simulink model "B737_PLANT"  (R2018a)
settings: Solver=VariableStepAuto  StartTime=0.0  StopTime=10.0  RelTol=1e-3
undefined symbols (not defined in the file): S
settings Model: Creator=Can Bekar  LastModifiedBy=Can Bekar
settings ModelReferenceCC: ModelReferenceNumInstancesAllowed=Single

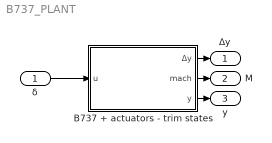
== system B737_PLANT ==
  δ : Inport
  B737 + actuators - trim states : Subsystem
  Δy : Outport
  M : Outport  Port=2
  y : Outport  Port=3
  wires:
  δ/1 -> B737 + actuators - trim states/1(u)
  B737 + actuators - trim states/2(mach) -> M/1
  B737 + actuators - trim states/1(Δy) -> Δy/1
  B737 + actuators - trim states/3(y) -> y/1

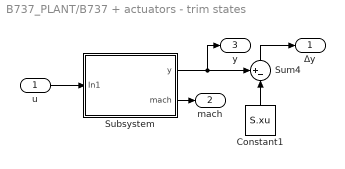
== system B737_PLANT/B737 + actuators - trim states ==
  u : Inport
  Constant1 : Constant  Value=S.xu
  Subsystem : Subsystem
  Sum4 : Sum  Inputs=+-|
  Δy : Outport
  mach : Outport  Port=2
  y : Outport  Port=3
  wires:
  Sum4/1 -> Δy/1
  Subsystem/1(y) -> y/1, Sum4/1
  u/1 -> Subsystem/1(In1)
  Constant1/1 -> Sum4/2
  Subsystem/2(mach) -> mach/1

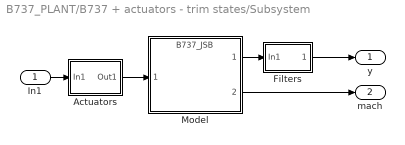
== system B737_PLANT/B737 + actuators - trim states/Subsystem ==
  In1 : Inport
  Actuators : Subsystem
  Filters : Subsystem
  Model : ModelReference  ModelNameDialog=B737_JSB.slx  SimulationMode=Normal  ModelReferenceVersion=1.187
  y : Outport
  mach : Outport  Port=2
  wires:
  Model/2 -> mach/1
  Model/1 -> Filters/1(In1)
  Filters/1(Out1) -> y/1
  In1/1 -> Actuators/1(In1)
  Actuators/1(Out1) -> Model/1

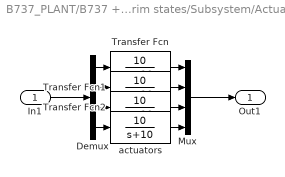
== system B737_PLANT/B737 + actuators - trim states/Subsystem/Actuators ==
  In1 : Inport
  Demux : Demux
  Mux : Mux
  Transfer Fcn : TransferFcn  Numerator=[10]  Denominator=[1 10]
  Transfer Fcn1 : TransferFcn  Numerator=[10]  Denominator=[1 10]
  Transfer Fcn2 : TransferFcn  Numerator=[10]  Denominator=[1 10]
  actuators : TransferFcn  Numerator=[10]  Denominator=[1 10]
  Out1 : Outport
  wires:
  actuators/1 -> Mux/4
  Transfer Fcn/1 -> Mux/1
  In1/1 -> Demux/1
  Demux/2 -> Transfer Fcn1/1
  Transfer Fcn1/1 -> Mux/2
  Demux/3 -> Transfer Fcn2/1
  Transfer Fcn2/1 -> Mux/3
  Demux/4 -> actuators/1
  Demux/1 -> Transfer Fcn/1
  Mux/1 -> Out1/1

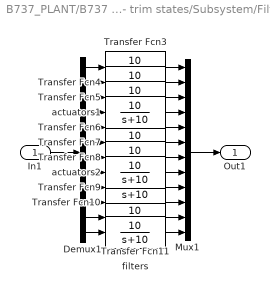
== system B737_PLANT/B737 + actuators - trim states/Subsystem/Filters ==
  In1 : Inport
  Demux1 : Demux  Outputs=12
  Mux1 : Mux  Inputs=12
  Transfer Fcn{3..11} (9 alike) : TransferFcn  Numerator=[10]  Denominator=[1 10]
  actuators1 : TransferFcn  Numerator=[10]  Denominator=[1 10]
  actuators2 : TransferFcn  Numerator=[10]  Denominator=[1 10]
  filters : TransferFcn  Numerator=[10]  Denominator=[1 10]
  Out1 : Outport
  wires:
  Demux1/11 -> Transfer Fcn11/1
  Transfer Fcn8/1 -> Mux1/7
  Transfer Fcn4/1 -> Mux1/2
  filters/1 -> Mux1/12
  Demux1/3 -> Transfer Fcn5/1
  Transfer Fcn7/1 -> Mux1/6
  Demux1/12 -> filters/1
  actuators1/1 -> Mux1/4
  Transfer Fcn3/1 -> Mux1/1
  Transfer Fcn11/1 -> Mux1/11
  In1/1 -> Demux1/1
  Demux1/9 -> Transfer Fcn9/1
  Transfer Fcn6/1 -> Mux1/5
  Demux1/1 -> Transfer Fcn3/1
  Demux1/4 -> actuators1/1
  Transfer Fcn5/1 -> Mux1/3
  Demux1/2 -> Transfer Fcn4/1
  Demux1/8 -> actuators2/1
  Transfer Fcn10/1 -> Mux1/10
  Demux1/10 -> Transfer Fcn10/1
  Transfer Fcn9/1 -> Mux1/9
  Demux1/5 -> Transfer Fcn6/1
  Demux1/6 -> Transfer Fcn7/1
  Demux1/7 -> Transfer Fcn8/1
  Mux1/1 -> Out1/1
  actuators2/1 -> Mux1/8
